simulink model "b2"  (R2020a)
settings: Solver=VariableStepAuto  StartTime=0.0  StopTime=10.0  RelTol=1e-3
libraries: simulink_need_slupdate x2, simulink x2
settings Model: Creator=Erfan  LastModifiedBy=Erfan

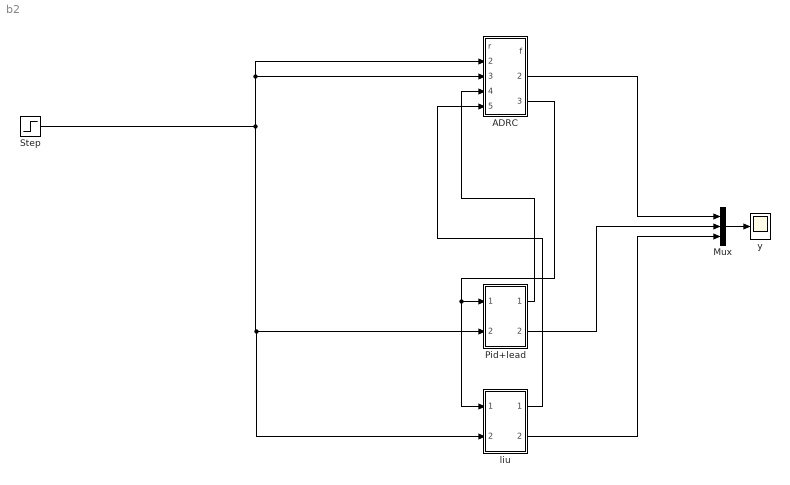
== system b2 ==
  ADRC : Subsystem
  Mux : Mux  Inputs=3
  Pid+lead : Subsystem
  Step : Step  SampleTime=0
  liu : Subsystem
  y : Scope
  wires:
  ADRC/3(Out3) -> liu/1(In1), Pid+lead/1(In1)
  Pid+lead/1(Out1) -> ADRC/4(In4)
  ADRC/2(Out2) -> Mux/1
  liu/2(Out2) -> Mux/3
  Pid+lead/2(Out2) -> Mux/2
  Step/1 -> ADRC/3(In3), ADRC/2(In2), liu/2(In2), Pid+lead/2(In2)
  liu/1(Out1) -> ADRC/5(In1)
  Mux/1 -> y/1

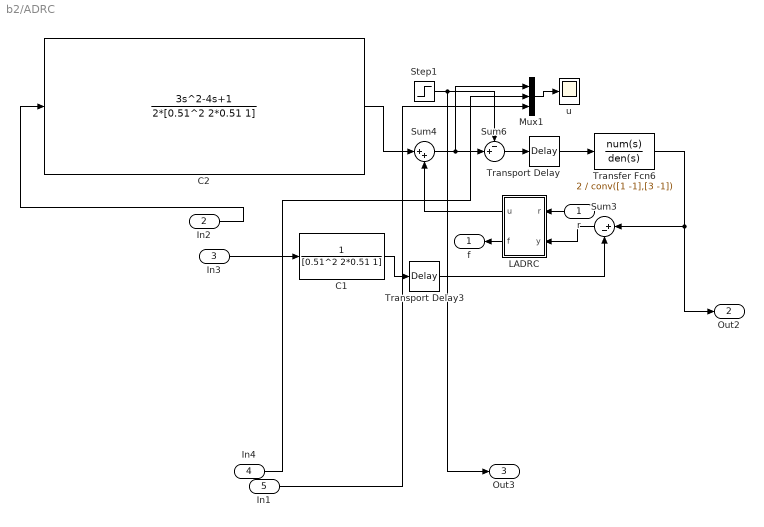
== system b2/ADRC ==
  r : Inport
  In2 : Inport  Port=2
  In3 : Inport  Port=3
  In4 : Inport  Port=4
  In1 : Inport  Port=5
  C1 : TransferFcn  Numerator=1  Denominator=[0.51^2 2*0.51 1]
  C2 : TransferFcn  Numerator=[3 -4 1]  Denominator=2*[0.51^2 2*0.51 1]
  LADRC : Subsystem  mask{n=3, b0=1, Ko=[61341.2837 2914.1104 92.2411 1], Lo=[0.4256;4.9673;2.9762;1.5846]}
      mask prompts: n "order"; b0 "high-frequency gain"; Ko "feedback gain"; Lo "observer gain"
  Mux1 : Mux  Inputs=3
  Step1 : Step  Time=20  SampleTime=0
  Sum3 : Sum  Inputs=|+-  SaturateOnIntegerOverflow=on
  Sum4 : Sum  Inputs=|++  SaturateOnIntegerOverflow=on
  Sum6 : Sum  Inputs=-+|  InputSameDT=on  SaturateOnIntegerOverflow=on  OutDataTypeStr=Inherit: Same as first input
  Transfer Fcn6 : TransferFcn  Numerator=2  Denominator=conv([1 -1],[3 -1])
  Transport Delay : TransportDelay  DelayTime=0.3
  Transport Delay3 : TransportDelay  DelayTime=0.3
  u : Scope
  f : Outport
  Out2 : Outport  Port=2
  Out3 : Outport  Port=3
  wires:
  Sum3/1 -> LADRC/2(y)
  C2/1 -> Sum4/1
  Transport Delay3/1 -> Sum3/2
  C1/1 -> Transport Delay3/1
  Sum6/1 -> Transport Delay/1
  Step1/1 -> Sum6/1, Out3/1
  Transport Delay/1 -> Transfer Fcn6/1
  Transfer Fcn6/1 -> Out2/1, Sum3/1
  LADRC/1(u) -> Sum4/2
  LADRC/2(f) -> f/1
  Sum4/1 -> Mux1/1, Sum6/2
  Mux1/1 -> u/1
  r/1 -> LADRC/1(r)
  In2/1 -> C2/1
  In3/1 -> C1/1
  In4/1 -> Mux1/2
  In1/1 -> Mux1/3

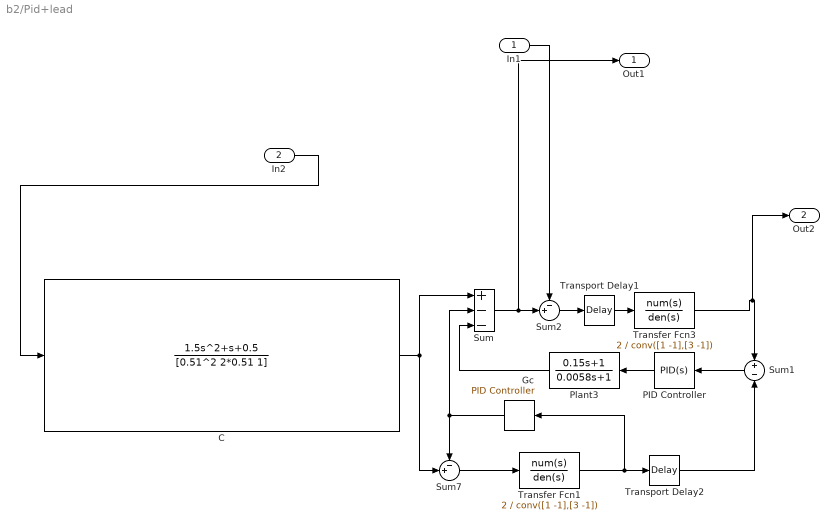
== system b2/Pid+lead ==
  In1 : Inport
  In2 : Inport  Port=2
  C : TransferFcn  Numerator=[1.5 1 0.5]  Denominator=[0.51^2 2*0.51 1]
  Gc : simulink_need_slupdate/PID Controller  P=0  I=0  D=3
  PID Controller : simulink/Continuous/PID Controller  Controller=PID  Form=Parallel  TimeDomain=Continuous-time  UseExternalTs=off  SampleTime=1  IntegratorMethod=Forward Euler  FilterMethod=Forward Euler  ControllerParametersSource=internal  P=3.5671  I=3.5671/1.491  D=3.5671*1.3364  UseFilter=on  N=100  TunerSelectOption=Transfer Function Based (PID Tuner App)  InitialConditionSource=internal  InitialConditionForIntegrator=0  InitialConditionForFilter=0  DifferentiatorICPrevScaledInput=0  ExternalReset=none  TrackingMode=off  Kt=1  LimitOutput=off  UpperSaturationLimit=inf  LowerSaturationLimit=-inf  LinearizeAsGain=on  AntiWindupMode=none  Kb=1  POutMin=[]  POutMax=[]  IOutMin=[]  IOutMax=[]  DOutMin=[]  DOutMax=[]  NOutMin=[]  NOutMax=[]  SumOutMin=[]  SumOutMax=[]  SaturationOutMin=[]  SaturationOutMax=[]  PParamMin=[]  PParamMax=[]  IParamMin=[]  IParamMax=[]  DParamMin=[]  DParamMax=[]  NParamMin=[]  NParamMax=[]  KbParamMin=[]  KbParamMax=[]  KtParamMin=[]  KtParamMax=[]  KbOutMin=[]  KbOutMax=[]  KtOutMin=[]  KtOutMax=[]  IntegratorOutMin=[]  IntegratorOutMax=[]  FilterOutMin=[]  FilterOutMax=[]  SumI1OutMin=[]  SumI1OutMax=[]  SumI2OutMin=[]  SumI2OutMax=[]  SumI3OutMin=[]  SumI3OutMax=[]  SumI4OutMin=[]  SumI4OutMax=[]  SumDOutMin=[]  SumDOutMax=[]  DifferentiatorOutMin=[]  DifferentiatorOutMax=[]  FilterDiffOutCoefMin=[]  FilterDiffOutCoefMax=[]  ReciprocalOutMin=[]  ReciprocalOutMax=[]  SumDenOutMin=[]  SumDenOutMax=[]  SumNumOutMin=[]  SumNumOutMax=[]  DivideOutMin=[]  DivideOutMax=[]  UdiffTsProdOutMin=[]  UdiffTsProdOutMax=[]  NTsProdOutMin=[]  NTsProdOutMax=[]  UintegralTsProdOutMin=[]  UintegralTsProdOutMax=[]  UngainTsProdOutMin=[]  UngainTsProdOutMax=[]  IntegratorContinuousStateAttributes=''  IntegratorStateMustResolveToSignalObject=off  IntegratorRTWStateStorageClass=Auto  FilterContinuousStateAttributes=''  FilterStateMustResolveToSignalObject=off  FilterRTWStateStorageClass=Auto  ParallelPVariant=InternalParameters  IdealPVariant=Disabled  IVariant=InternalParameters  DVariant=InternalParameters  IntegratorVariant=Continuous  SatVariant=Disabled  AWVariant=Passthrough  PCopyVariant=Disabled  TRVariant=Disabled  FdbkBlocksVariant=Forward  IdealPFdbkVariant=Disabled  SatFdbkVariant=Disabled  DerivativeFilterVariant=ContFilter  NVariant=InternalParameters  NCopyVariant=Disabled  FilterICVariant=InternalICsFilter  IntegratorICVariant=InternalICs  ExternalResetVariant=Disabled  TRSumVariant=Passthrough  SumFdbkVariant=Disabled  SumVariant=Sum_PID  TsampFilterVariant=InternalTs  TsampNgainVariant=Passthrough  TsampIntegralVariant=Passthrough
  Plant3 : TransferFcn  Numerator=[0.15 1]  Denominator=[0.0058 1]
  Sum : Sum  Inputs=+--  SaturateOnIntegerOverflow=on
  Sum1 : Sum  Inputs=+|-  SaturateOnIntegerOverflow=on
  Sum2 : Sum  Inputs=-+|  SaturateOnIntegerOverflow=on
  Sum7 : Sum  Inputs=-+|  SaturateOnIntegerOverflow=on
  Transfer Fcn1 : TransferFcn  Numerator=2  Denominator=conv([1 -1],[3 -1])
  Transfer Fcn3 : TransferFcn  Numerator=2  Denominator=conv([1 -1],[3 -1])
  Transport Delay1 : TransportDelay  DelayTime=0.3
  Transport Delay2 : TransportDelay  DelayTime=0.3
  Out1 : Outport
  Out2 : Outport  Port=2
  wires:
  Sum/1 -> Out1/1, Sum2/2
  Transport Delay2/1 -> Sum1/2
  Transfer Fcn3/1 -> Out2/1, Sum1/1
  C/1 -> Sum/1, Sum7/2
  Gc/1 -> Sum/2, Sum7/1
  Sum1/1 -> PID Controller/1
  Sum7/1 -> Transfer Fcn1/1
  Transport Delay1/1 -> Transfer Fcn3/1
  PID Controller/1 -> Plant3/1
  Transfer Fcn1/1 -> Gc/1, Transport Delay2/1
  Plant3/1 -> Sum/3
  Sum2/1 -> Transport Delay1/1
  In2/1 -> C/1
  In1/1 -> Sum2/1

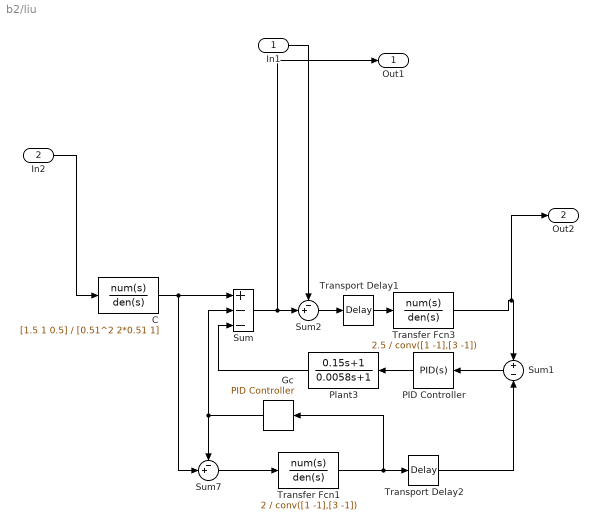
== system b2/liu ==
  In1 : Inport
  In2 : Inport  Port=2
  C : TransferFcn  Numerator=[1.5 1 0.5]  Denominator=[0.51^2 2*0.51 1]
  Gc : simulink_need_slupdate/PID Controller  P=0  I=0  D=3
  PID Controller : simulink/Continuous/PID Controller  Controller=PID  Form=Parallel  TimeDomain=Continuous-time  UseExternalTs=off  SampleTime=1  IntegratorMethod=Forward Euler  FilterMethod=Forward Euler  ControllerParametersSource=internal  P=3.5671  I=3.5671/1.491  D=3.5671*1.3364  UseFilter=on  N=100  TunerSelectOption=Transfer Function Based (PID Tuner App)  InitialConditionSource=internal  InitialConditionForIntegrator=0  InitialConditionForFilter=0  DifferentiatorICPrevScaledInput=0  ExternalReset=none  TrackingMode=off  Kt=1  LimitOutput=off  UpperSaturationLimit=inf  LowerSaturationLimit=-inf  LinearizeAsGain=on  AntiWindupMode=none  Kb=1  POutMin=[]  POutMax=[]  IOutMin=[]  IOutMax=[]  DOutMin=[]  DOutMax=[]  NOutMin=[]  NOutMax=[]  SumOutMin=[]  SumOutMax=[]  SaturationOutMin=[]  SaturationOutMax=[]  PParamMin=[]  PParamMax=[]  IParamMin=[]  IParamMax=[]  DParamMin=[]  DParamMax=[]  NParamMin=[]  NParamMax=[]  KbParamMin=[]  KbParamMax=[]  KtParamMin=[]  KtParamMax=[]  KbOutMin=[]  KbOutMax=[]  KtOutMin=[]  KtOutMax=[]  IntegratorOutMin=[]  IntegratorOutMax=[]  FilterOutMin=[]  FilterOutMax=[]  SumI1OutMin=[]  SumI1OutMax=[]  SumI2OutMin=[]  SumI2OutMax=[]  SumI3OutMin=[]  SumI3OutMax=[]  SumI4OutMin=[]  SumI4OutMax=[]  SumDOutMin=[]  SumDOutMax=[]  DifferentiatorOutMin=[]  DifferentiatorOutMax=[]  FilterDiffOutCoefMin=[]  FilterDiffOutCoefMax=[]  ReciprocalOutMin=[]  ReciprocalOutMax=[]  SumDenOutMin=[]  SumDenOutMax=[]  SumNumOutMin=[]  SumNumOutMax=[]  DivideOutMin=[]  DivideOutMax=[]  UdiffTsProdOutMin=[]  UdiffTsProdOutMax=[]  NTsProdOutMin=[]  NTsProdOutMax=[]  UintegralTsProdOutMin=[]  UintegralTsProdOutMax=[]  UngainTsProdOutMin=[]  UngainTsProdOutMax=[]  IntegratorContinuousStateAttributes=''  IntegratorStateMustResolveToSignalObject=off  IntegratorRTWStateStorageClass=Auto  FilterContinuousStateAttributes=''  FilterStateMustResolveToSignalObject=off  FilterRTWStateStorageClass=Auto  ParallelPVariant=InternalParameters  IdealPVariant=Disabled  IVariant=InternalParameters  DVariant=InternalParameters  IntegratorVariant=Continuous  SatVariant=Disabled  AWVariant=Passthrough  PCopyVariant=Disabled  TRVariant=Disabled  FdbkBlocksVariant=Forward  IdealPFdbkVariant=Disabled  SatFdbkVariant=Disabled  DerivativeFilterVariant=ContFilter  NVariant=InternalParameters  NCopyVariant=Disabled  FilterICVariant=InternalICsFilter  IntegratorICVariant=InternalICs  ExternalResetVariant=Disabled  TRSumVariant=Passthrough  SumFdbkVariant=Disabled  SumVariant=Sum_PID  TsampFilterVariant=InternalTs  TsampNgainVariant=Passthrough  TsampIntegralVariant=Passthrough
  Plant3 : TransferFcn  Numerator=[0.15 1]  Denominator=[0.0058 1]
  Sum : Sum  Inputs=+--  SaturateOnIntegerOverflow=on
  Sum1 : Sum  Inputs=+|-  SaturateOnIntegerOverflow=on
  Sum2 : Sum  Inputs=-+|  SaturateOnIntegerOverflow=on
  Sum7 : Sum  Inputs=-+|  SaturateOnIntegerOverflow=on
  Transfer Fcn1 : TransferFcn  Numerator=2  Denominator=conv([1 -1],[3 -1])
  Transfer Fcn3 : TransferFcn  Numerator=2.5  Denominator=conv([1 -1],[3 -1])
  Transport Delay1 : TransportDelay  DelayTime=0.3
  Transport Delay2 : TransportDelay  DelayTime=0.3
  Out1 : Outport
  Out2 : Outport  Port=2
  wires:
  Sum/1 -> Out1/1, Sum2/2
  Transport Delay2/1 -> Sum1/2
  Transfer Fcn3/1 -> Out2/1, Sum1/1
  C/1 -> Sum7/2, Sum/1
  Gc/1 -> Sum/2, Sum7/1
  Sum1/1 -> PID Controller/1
  Sum7/1 -> Transfer Fcn1/1
  Transport Delay1/1 -> Transfer Fcn3/1
  PID Controller/1 -> Plant3/1
  Transfer Fcn1/1 -> Gc/1, Transport Delay2/1
  Plant3/1 -> Sum/3
  Sum2/1 -> Transport Delay1/1
  In2/1 -> C/1
  In1/1 -> Sum2/1

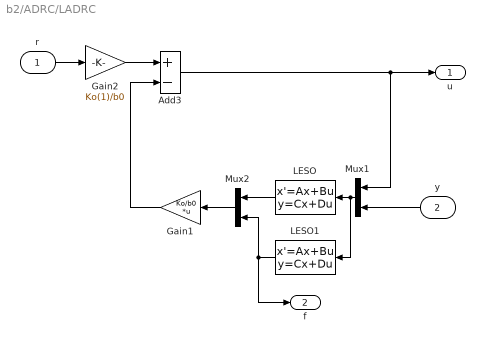
== system b2/ADRC/LADRC ==
  r : Inport
  y : Inport  Port=2
  Add3 : Sum  Inputs=+-
  Gain1 : Gain  Gain=Ko/b0  Multiplication=Matrix(K*u)
  Gain2 : Gain  Gain=Ko(1)/b0
  LESO : StateSpace  A=[zeros(n,1) eye(n,n);zeros(1,n+1)]-Lo*[1 zeros(1,n)]  B=[[zeros(n-1,1);b0;0] Lo]  C=[eye(n,n) zeros(n,1)]  D=zeros(n,2)  InitialCondition=0
  LESO1 : StateSpace  A=[zeros(n,1) eye(n,n);zeros(1,n+1)]-Lo*[1 zeros(1,n)]  B=[[zeros(n-1,1);b0;0] Lo]  C=[zeros(1,n) 1]  D=[0 0]  InitialCondition=0
  Mux1 : Mux  Inputs=2
  Mux2 : Mux  Inputs=2
  u : Outport
  f : Outport  Port=2
  wires:
  Gain1/1 -> Add3/2
  LESO1/1 -> Mux2/2, f/1
  Mux2/1 -> Gain1/1
  LESO/1 -> Mux2/1
  r/1 -> Gain2/1
  Mux1/1 -> LESO/1, LESO1/1
  y/1 -> Mux1/2
  Add3/1 -> Mux1/1, u/1
  Gain2/1 -> Add3/1
